simulink model "obserwator_regulator_na_obiekcie"  (R2017b)
settings: Solver=VariableStepAuto  StartTime=0.0  StopTime=5  RelTol=1e-3
values from neighbouring files (symbols this model uses):
  A = [3.22791678547  1  0; -1.44925930399  0  1; 0.17377394345  0  0]    [matlab.mat]
  A2 = [3.22791678547  1  0; -1.44925930399  0  1; 0.17377394345  0  0]    [matlab.mat]
  B = [0.260707487539 -0.289205764977 0.0761198486843]    [matlab.mat]
  B2 = [0.260707487539 -0.289205764977 0.0761198486843]    [matlab.mat]
  K = [11.2993624638 4.84519726655 2.40866701447]    [matlab.mat]
  L = [-1 0.25]    [matlab.mat]
  Tp = 0.25    [matlab.mat]
  x_start = [3 -2 1]    [matlab.mat]
settings Model: Creator=gulin  LastModifiedBy=gulin

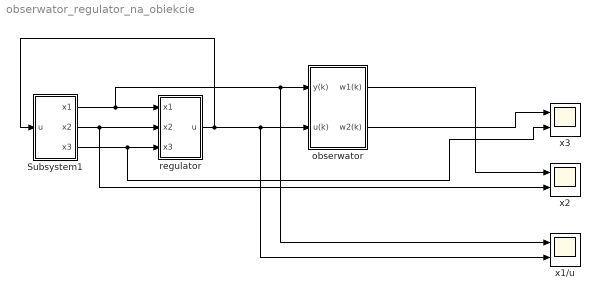
== system obserwator_regulator_na_obiekcie ==
  Subsystem1 : Subsystem
  "obserwator " : Subsystem
  regulator : Subsystem
  x1/u : Scope  NumInputPorts=2
  x2 : Scope  NumInputPorts=2
  x3 : Scope  NumInputPorts=2
  wires:
  Subsystem1/1(x1) -> x1/u/1, "obserwator "/1(y(k)), regulator/1(x1)
  Subsystem1/2(x2) -> x2/2, regulator/2(x2)
  Subsystem1/3(x3) -> x3/2, regulator/3(x3)
  regulator/1("u ") -> x1/u/2, "obserwator "/2("u(k) "), Subsystem1/1("u ")
  "obserwator "/1(w1(k)) -> x2/1
  "obserwator "/2(w2(k)) -> x3/1

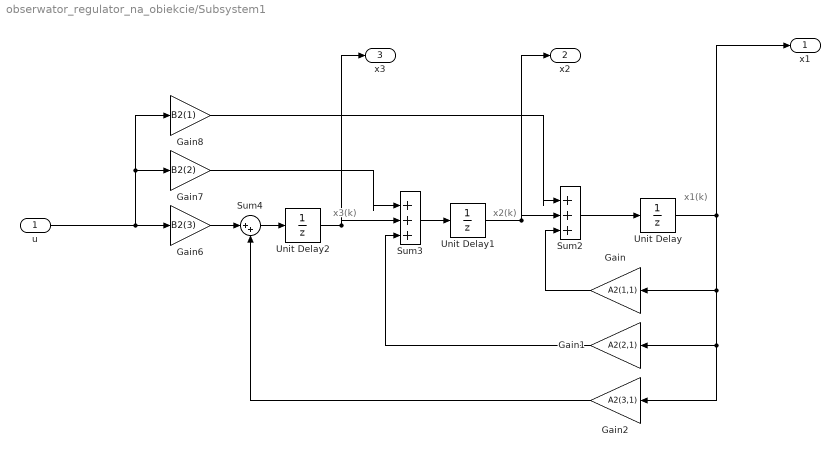
== system obserwator_regulator_na_obiekcie/Subsystem1 ==
  note: x1(k)
  note: x3(k)
  note: x2(k)
  "u " : Inport
  Gain : Gain  Gain=A2(1,1)
  Gain1 : Gain  Gain=A2(2,1)
  Gain2 : Gain  Gain=A2(3,1)
  Gain6 : Gain  Gain=B2(3)
  Gain7 : Gain  Gain=B2(2)
  Gain8 : Gain  Gain=B2(1)
  Sum2 : Sum  Inputs=|+++
  Sum3 : Sum  Inputs=|+++
  Sum4 : Sum  Inputs=|++
  Unit Delay : UnitDelay  InitialCondition=x_start(1)  SampleTime=Tp
  Unit Delay1 : UnitDelay  InitialCondition=x_start(2)  SampleTime=Tp
  Unit Delay2 : UnitDelay  InitialCondition=x_start(3)  SampleTime=Tp
  x1 : Outport
  x2 : Outport  Port=2
  x3 : Outport  Port=3
  wires:
  Unit Delay/1 -> Gain2/1, Gain1/1, Gain/1, x1/1
  Sum2/1 -> Unit Delay/1
  Gain2/1 -> Sum4/2
  Gain1/1 -> Sum3/3
  Sum4/1 -> Unit Delay2/1
  Gain6/1 -> Sum4/1
  Unit Delay2/1 -> Sum3/2, x3/1
  Gain/1 -> Sum2/3
  Gain8/1 -> Sum2/1
  Sum3/1 -> Unit Delay1/1
  Unit Delay1/1 -> x2/1, Sum2/2
  Gain7/1 -> Sum3/1
  "u "/1 -> Gain8/1, Gain7/1, Gain6/1

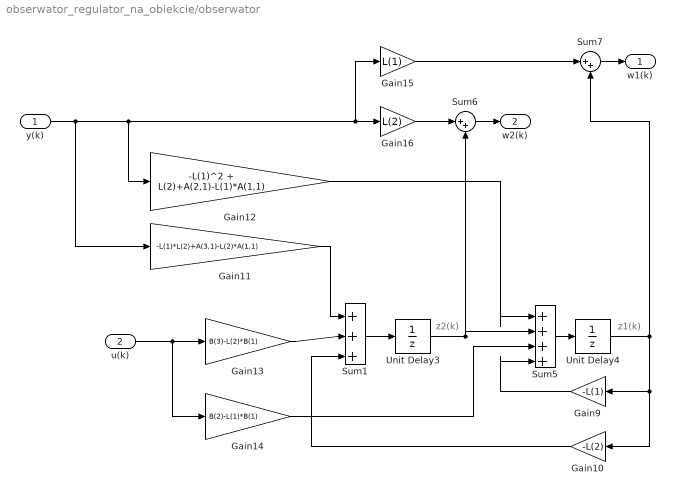
== system obserwator_regulator_na_obiekcie/obserwator  ==
  note: z1(k)
  note: z2(k)
  y(k) : Inport
  "u(k) " : Inport  Port=2
  Gain10 : Gain  Gain=-L(2)
  Gain11 : Gain  Gain=-L(1)*L(2)+A(3,1)-L(2)*A(1,1)
  Gain12 : Gain  Gain=-L(1)^2 + L(2)+A(2,1)-L(1)*A(1,1)
  Gain13 : Gain  Gain=B(3)-L(2)*B(1)
  Gain14 : Gain  Gain=B(2)-L(1)*B(1)
  Gain15 : Gain  Gain=L(1)
  Gain16 : Gain  Gain=L(2)
  Gain9 : Gain  Gain=-L(1)
  Sum1 : Sum  Inputs=|+++
  Sum5 : Sum  Inputs=|++++
  Sum6 : Sum  Inputs=|++
  Sum7 : Sum  Inputs=|++
  Unit Delay3 : UnitDelay  SampleTime=Tp
  Unit Delay4 : UnitDelay  SampleTime=Tp
  w1(k) : Outport
  w2(k) : Outport  Port=2
  wires:
  Gain9/1 -> Sum5/4
  Gain16/1 -> Sum6/1
  Unit Delay4/1 -> Gain10/1, Gain9/1, Sum7/2
  Gain14/1 -> Sum5/3
  Sum1/1 -> Unit Delay3/1
  Gain11/1 -> Sum1/1
  Gain15/1 -> Sum7/1
  Gain10/1 -> Sum1/3
  Gain13/1 -> Sum1/2
  Gain12/1 -> Sum5/1
  Unit Delay3/1 -> Sum5/2, Sum6/2
  Sum5/1 -> Unit Delay4/1
  Sum6/1 -> w2(k)/1
  "u(k) "/1 -> Gain14/1, Gain13/1
  Sum7/1 -> w1(k)/1
  y(k)/1 -> Gain15/1, Gain16/1, Gain12/1, Gain11/1

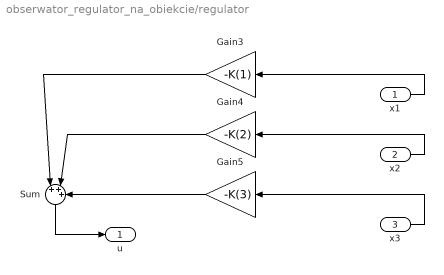
== system obserwator_regulator_na_obiekcie/regulator ==
  x1 : Inport
  x2 : Inport  Port=2
  x3 : Inport  Port=3
  Gain3 : Gain  Gain=-K(1)
  Gain4 : Gain  Gain=-K(2)
  Gain5 : Gain  Gain=-K(3)
  Sum : Sum  Inputs=|+++
  "u " : Outport
  wires:
  Gain4/1 -> Sum/2
  Gain5/1 -> Sum/3
  Sum/1 -> "u "/1
  Gain3/1 -> Sum/1
  x3/1 -> Gain5/1
  x2/1 -> Gain4/1
  x1/1 -> Gain3/1
